simulink model "sm_DynamicCompression"  (R2019b)
settings: Solver=FixedStepDiscrete  StartTime=0.0  StopTime=stop_time  RelTol=1e-3
InitFcn:
  | sm_callback_init
StopFcn:
  | sm_callback_stop
values from neighbouring files (symbols this model uses):
  a = 100*(r^2)    [InitializeCompressionSettings.m]    (also in sm_check_control_signals.m = registers(i).(supplied_fields{j}); sm_check_control_signals_LOCAL_1434.m = registers(i).(supplied_fields{j}))
  B_k_0_init = zeros(1,FIR_0_Uprate)    [sm_callback_init.m]
  B_k_1_init = zeros(1,FIR_0_Uprate)    [sm_callback_init.m]
  B_k_2_init = zeros(1,FIR_0_Uprate)    [sm_callback_init.m]
  B_k_3_init = zeros(1,FIR_0_Uprate)    [sm_callback_init.m]
  B_k_4_init = zeros(1,FIR_0_Uprate)    [sm_callback_init.m]
  B_k_5_init = zeros(1,FIR_0_Uprate)    [sm_callback_init.m]
  calib_bpfs = bpfs    [sm_compression_init.m]
  delayFix = maxDelay-delays    [Initialize_Delay_Values.m]
  F_bits = 28    [TestingLibraryScripts.m]    (also in sm_compression_init.m)
  FIR_0_Size = (ceil(log2(length(calib_bpfs(2:calib_bpfs(1,1)+1 ,1)'))))    [sm_callback_init.m]
  FIR_0_Uprate = 2^FIR_0_Size    [sm_callback_init.m]
  M_bits = 1    [TestingLibraryScripts.m]    (also in sm_compression_init.m = 5)
  M_Bits = M_bits    (= 5)    [sm_compression_init.m]
  mp = sm_init_avalon_signals(mp)    [sm_callback_init.m]
  r_att = nthroot(0.1, s_att)    [sm_compression_init.m]
  r_rel = nthroot(0.1, s_rel)    [sm_compression_init.m]
  recombGain = ones(1,NChans)    [sm_compression_init.m]
  TABLE_SEL_BYPASS_ENABLE = 0    [sm_callback_init.m]
  Ts = mp.Ts    [sm_compression_init.m]
  Ts_system = mp.Ts_system    [sm_compression_init.m]
  W_bits = 32    [TestingLibraryScripts.m]    (also in sm_compression_init.m)
  X_high = 1    [sm_compression_init.m]
undefined symbols (not defined in the file or in its folder): b, c, Gain_Table, ig_eq
libraries: hdlsllib x272, simulink x127, dsphdlfiltering x2
(part 7 of 8)

== matlab function sm_DynamicCompression/dataplane/Avalon Data Processing/Left Channel Processing/recalculate/Nchan_FbankAGC_AID/Compression_1/Compression_Gain_Calc/LogAddressing/MATLAB Function ==
  data: x input; lzc_count output
function lzc_count = fcn(x)
%#codegen

% -- Binary Bisection Tree (Divide & Conquer)
if bitorreduce(x, 40, 21) == 1 %       if ((b39 or b38 or b37 or b36 or b35 or b34 or b33 or b32 or b31 or b30 or b29 or b28 or b27 or b26 or b25 or b24 or b23 or b22 or b21 or b20) = '1') then   -- check bit range [39  20]
    if bitorreduce(x, 40, 31) == 1%             if ((b39 or b38 or b37 or b36 or b35 or b34 or b33 or b32 or b31 or b30) = '1') then   -- check bit range [39  30]
        if bitorreduce(x, 40, 36) == 1%                 if ((b39 or b38 or b37 or b36 or b35) = '1') then   -- check bit range [39  35]
            if bitorreduce(x, 40, 38) == 1%                     if ((b39 or b38 or b37) = '1') then   -- check bit range [39  37]
                if bitorreduce(x, 40, 39) == 1%                         if ((b39 or b38) = '1') then   -- check bit range [39  38]
                    if bitorreduce(x, 40, 40) == 1%                             if (b39 = '1') then   -- [39]
                        lzc_count = fi(0,0,6,0);%                                 lzc_count <= "000000";  -- lzc = 0
                    else%                             else  -- check bit range [38]
                        lzc_count = fi(1,0,6,0);%                                 lzc_count <= "000001";  -- lzc = 1
                    end%                             end if;
                else%                         else  -- check bit range [37]
                    lzc_count = fi(2,0,6,0);%                             lzc_count <= "000010";  -- lzc = 2
                end%                         end if;
            else%                     else  -- check bit range [36  35]
                if bitorreduce(x, 37, 37) == 1%                         if (b36 = '1') then   -- [36]
                    lzc_count = fi(3,0,6,0);%                             lzc_count <= "000011";  -- lzc = 3
                else%                         else  -- check bit range [35]
                    lzc_count = fi(4,0,6,0);%                             lzc_count <= "000100";  -- lzc = 4
                end%                         end if;
            end%                     end if;
        else%                 else  -- check bit range [34  30]
            if bitorreduce(x, 35, 33) == 1%                     if ((b34 or b33 or b32) = '1') then   -- check bit range [34  32]
                if bitorreduce(x, 35, 34) == 1%                         if ((b34 or b33) = '1') then   -- check bit range [34  33]
                    if bitorreduce(x, 35, 35) == 1%                             if (b34 = '1') then   -- [34]
                        lzc_count = fi(5,0,6,0);%                                 lzc_count <= "000101";  -- lzc = 5
                    else%                             else  -- check bit range [33]
                        lzc_count = fi(6,0,6,0);%                                 lzc_count <= "000110";  -- lzc = 6
                    end%                             end if;
                else%                         else  -- check bit range [32]
                    lzc_count = fi(7,0,6,0);%                             lzc_count <= "000111";  -- lzc = 7
                end%                         end if;
            else%                     else  -- check bit range [31  30]
                if bitorreduce(x, 32, 32) == 1%                         if (b31 = '1') then   -- [31]
                    lzc_count = fi(8,0,6,0);%                             lzc_count <= "001000";  -- lzc = 8
                else%                         else  -- check bit range [30]
                    lzc_count = fi(9,0,6,0);%                             lzc_count <= "001001";  -- lzc = 9
                end%                         end if;
            end%                     end if;
        end%                 end if;
    else%             else  -- check bit range [29  20]
        if bitorreduce(x, 30, 26) == 1%                 if ((b29 or b28 or b27 or b26 or b25) = '1') then   -- check bit range [29  25]
            if bitorreduce(x, 30, 28) == 1%                     if ((b29 or b28 or b27) = '1') then   -- check bit range [29  27]
                if bitorreduce(x, 30, 29) == 1%                         if ((b29 or b28) = '1') then   -- check bit range [29  28]
                    if bitorreduce(x, 30, 30) == 1%                             if (b29 = '1') then   -- [29]
                        lzc_count = fi(10,0,6,0);%                                 lzc_count <= "001010";  -- lzc = 10
                    else%                             else  -- check bit range [28]
                        lzc_count = fi(11,0,6,0);%                                 lzc_count <= "001011";  -- lzc = 11
                    end%                             end if;
                else%                         else  -- check bit range [27]
                    lzc_count = fi(12,0,6,0);%                             lzc_count <= "001100";  -- lzc = 12
                end%                         end if;
            else%                     else  -- check bit range [26  25]
                if bitorreduce(x, 27, 27) == 1%                         if (b26 = '1') then   -- [26]
                    lzc_count = fi(13,0,6,0);%                             lzc_count <= "001101";  -- lzc = 13
                else%                         else  -- check bit range [25]
                    lzc_count = fi(14,0,6,0);%                             lzc_count <= "001110";  -- lzc = 14
                end%                         end if;
            end%                     end if;
        else%                 else  -- check bit range [24  20]
            if bitorreduce(x, 25, 23) == 1%                     if ((b24 or b23 or b22) = '1') then   -- check bit range [24  22]
                if bitorreduce(x, 25, 24) == 1%                         if ((b24 or b23) = '1') then   -- check bit range [24  23]
                    if bitorreduce(x, 25, 25) == 1%                             if (b24 = '1') then   -- [24]
                        lzc_count = fi(15,0,6,0);%                                 lzc_count <= "001111";  -- lzc = 15
                    else%                             else  -- check bit range [23]
                        lzc_count = fi(16,0,6,0);%                                 lzc_count <= "010000";  -- lzc = 16
                    end%                             end if;
                else%                         else  -- check bit range [22]
                    lzc_count = fi(17,0,6,0);%                             lzc_count <= "010001";  -- lzc = 17
                end%                         end if;
            else%                     else  -- check bit range [21  20]
                if bitorreduce(x, 22, 22) == 1%                         if (b21 = '1') then   -- [21]
                    lzc_count = fi(18,0,6,0);%                             lzc_count <= "010010";  -- lzc = 18
                else%                         else  -- check bit range [20]
                    lzc_count = fi(19,0,6,0);%                             lzc_count <= "010011";  -- lzc = 19
                end%                         end if;
            end%                     end if;
        end%                 end if;
    end%             end if;
else%         else  -- check bit range [19   0]
    if bitorreduce(x, 20, 11) == 1%             if ((b19 or b18 or b17 or b16 or b15 or b14 or b13 or b12 or b11 or b10) = '1') then   -- check bit range [19  10]
        if bitorreduce(x, 20, 16) == 1%                 if ((b19 or b18 or b17 or b16 or b15) = '1') then   -- check bit range [19  15]
            if bitorreduce(x, 20, 18) == 1%                     if ((b19 or b18 or b17) = '1') then   -- check bit range [19  17]
                if bitorreduce(x, 20, 19) == 1%                         if ((b19 or b18) = '1') then   -- check bit range [19  18]
                    if bitorreduce(x, 20, 20) == 1%                             if (b19 = '1') then   -- [19]
                        lzc_count = fi(20,0,6,0);%                                 lzc_count <= "010100";  -- lzc = 20
                    else%                             else  -- check bit range [18]
                        lzc_count = fi(21,0,6,0);%                                 lzc_count <= "010101";  -- lzc = 21
                    end%                             end if;
                else%                         else  -- check bit range [17]
                    lzc_count = fi(22,0,6,0);%                             lzc_count <= "010110";  -- lzc = 22
                end%                         end if;
            else%                     else  -- check bit range [16  15]
                if bitorreduce(x, 17, 17) == 1%                         if (b16 = '1') then   -- [16]
                    lzc_count = fi(23,0,6,0);%                             lzc_count <= "010111";  -- lzc = 23
                else%                         else  -- check bit range [15]
                    lzc_count = fi(24,0,6,0);%                             lzc_count <= "011000";  -- lzc = 24
                end%                         end if;
            end%                     end if;
        else%                 else  -- check bit range [14  10]
            if bitorreduce(x, 15, 13) == 1%                     if ((b14 or b13 or b12) = '1') then   -- check bit range [14  12]
                if bitorreduce(x, 15, 14) == 1%                         if ((b14 or b13) = '1') then   -- check bit range [14  13]
                    if bitorreduce(x, 15, 15) == 1%                             if (b14 = '1') then   -- [14]
                        lzc_count = fi(25,0,6,0);%                                 lzc_count <= "011001";  -- lzc = 25
                    else%                             else  -- check bit range [13]
                        lzc_count = fi(26,0,6,0);%                                 lzc_count <= "011010";  -- lzc = 26
                    end%                             end if;
                else%                         else  -- check bit range [12]
                    lzc_count = fi(27,0,6,0);%                             lzc_count <= "011011";  -- lzc = 27
                end%                         end if;
            else%                     else  -- check bit range [11  10]
                if bitorreduce(x, 12, 12) == 1%                         if (b11 = '1') then   -- [11]
                    lzc_count = fi(28,0,6,0);%                             lzc_count <= "011100";  -- lzc = 28
                else%                         else  -- check bit range [10]
                    lzc_count = fi(29,0,6,0);%                             lzc_count <= "011101";  -- lzc = 29
                end%                         end if;
            end%                     end if;
        end%                 end if;
    else%             else  -- check bit range [9  0]
        if bitorreduce(x, 10, 6) == 1%                 if ((b9 or b8 or b7 or b6 or b5) = '1') then   -- check bit range [9  5]
            if bitorreduce(x, 10, 9) == 1%                     if ((b9 or b8 or b7) = '1') then   -- check bit range [9  7]
                if bitorreduce(x, 10, 9) == 1%                         if ((b9 or b8) = '1') then   -- check bit range [9  8]
                    if bitorreduce(x, 10, 10) == 1%                             if (b9 = '1') then   -- [9]
                        lzc_count = fi(30,0,6,0);%                                 lzc_count <= "011110";  -- lzc = 30
                    else%                             else  -- check bit range [8]
                        lzc_count = fi(31,0,6,0);%                                 lzc_count <= "011111";  -- lzc = 31
                    end%                             end if;
                else%                         else  -- check bit range [7]
                    lzc_count = fi(32,0,6,0);%                             lzc_count <= "100000";  -- lzc = 32
                end%                         end if;
            else%                     else  -- check bit range [6  5]
                if bitorreduce(x, 7, 7) == 1%                         if (b6 = '1') then   -- [6]
                    lzc_count = fi(33,0,6,0);%                             lzc_count <= "100001";  -- lzc = 33
                else%                         else  -- check bit range [5]
                    lzc_count = fi(34,0,6,0);%                             lzc_count <= "100010";  -- lzc = 34
                end%                         end if;
            end%                     end if;
        else%                 else  -- check bit range [4  0]
            if bitorreduce(x, 5, 3) == 1%                     if ((b4 or b3 or b2) = '1') then   -- check bit range [4  2]
                if bitorreduce(x, 5, 4) == 1%                         if ((b4 or b3) = '1') then   -- check bit range [4  3]
                    if bitorreduce(x, 5, 5) == 1%                             if (b4 = '1') then   -- [4]
                        lzc_count = fi(35,0,6,0);%                                 lzc_count <= "100011";  -- lzc = 35
                    else%                             else  -- check bit range [3]
                        lzc_count = fi(36,0,6,0);%                                 lzc_count <= "100100";  -- lzc = 36
                    end%                             end if;
                else%                         else  -- check bit range [2]
                    lzc_count = fi(37,0,6,0);%                             lzc_count <= "100101";  -- lzc = 37
                end%                         end if;
            else%                     else  -- check bit range [1  0]
                if bitorreduce(x, 2, 2) == 1%                         if (b1 = '1') then   -- [1]
                    lzc_count = fi(38,0,6,0);%                             lzc_count <= "100110";  -- lzc = 38
                else%                         else  -- check bit range [0]
                    lzc_count = fi(39,0,6,0);%                             lzc_count <= "100111";  -- lzc = 39
                end%                         end if;
            end%                     end if;
        end%                 end if;
    end%             end if;
end%         end if;

== matlab function sm_DynamicCompression/dataplane/Avalon Data Processing/Left Channel Processing/recalculate/Nchan_FbankAGC_AID/Compression_3/Compression_Gain_Calc/LogAddressing/MATLAB Function ==
  data: x input; lzc_count output
function lzc_count = fcn(x)
%#codegen

% -- Binary Bisection Tree (Divide & Conquer)
if bitorreduce(x, 40, 21) == 1 %       if ((b39 or b38 or b37 or b36 or b35 or b34 or b33 or b32 or b31 or b30 or b29 or b28 or b27 or b26 or b25 or b24 or b23 or b22 or b21 or b20) = '1') then   -- check bit range [39  20]
    if bitorreduce(x, 40, 31) == 1%             if ((b39 or b38 or b37 or b36 or b35 or b34 or b33 or b32 or b31 or b30) = '1') then   -- check bit range [39  30]
        if bitorreduce(x, 40, 36) == 1%                 if ((b39 or b38 or b37 or b36 or b35) = '1') then   -- check bit range [39  35]
            if bitorreduce(x, 40, 38) == 1%                     if ((b39 or b38 or b37) = '1') then   -- check bit range [39  37]
                if bitorreduce(x, 40, 39) == 1%                         if ((b39 or b38) = '1') then   -- check bit range [39  38]
                    if bitorreduce(x, 40, 40) == 1%                             if (b39 = '1') then   -- [39]
                        lzc_count = fi(0,0,6,0);%                                 lzc_count <= "000000";  -- lzc = 0
                    else%                             else  -- check bit range [38]
                        lzc_count = fi(1,0,6,0);%                                 lzc_count <= "000001";  -- lzc = 1
                    end%                             end if;
                else%                         else  -- check bit range [37]
                    lzc_count = fi(2,0,6,0);%                             lzc_count <= "000010";  -- lzc = 2
                end%                         end if;
            else%                     else  -- check bit range [36  35]
                if bitorreduce(x, 37, 37) == 1%                         if (b36 = '1') then   -- [36]
                    lzc_count = fi(3,0,6,0);%                             lzc_count <= "000011";  -- lzc = 3
                else%                         else  -- check bit range [35]
                    lzc_count = fi(4,0,6,0);%                             lzc_count <= "000100";  -- lzc = 4
                end%                         end if;
            end%                     end if;
        else%                 else  -- check bit range [34  30]
            if bitorreduce(x, 35, 33) == 1%                     if ((b34 or b33 or b32) = '1') then   -- check bit range [34  32]
                if bitorreduce(x, 35, 34) == 1%                         if ((b34 or b33) = '1') then   -- check bit range [34  33]
                    if bitorreduce(x, 35, 35) == 1%                             if (b34 = '1') then   -- [34]
                        lzc_count = fi(5,0,6,0);%                                 lzc_count <= "000101";  -- lzc = 5
                    else%                             else  -- check bit range [33]
                        lzc_count = fi(6,0,6,0);%                                 lzc_count <= "000110";  -- lzc = 6
                    end%                             end if;
                else%                         else  -- check bit range [32]
                    lzc_count = fi(7,0,6,0);%                             lzc_count <= "000111";  -- lzc = 7
                end%                         end if;
            else%                     else  -- check bit range [31  30]
                if bitorreduce(x, 32, 32) == 1%                         if (b31 = '1') then   -- [31]
                    lzc_count = fi(8,0,6,0);%                             lzc_count <= "001000";  -- lzc = 8
                else%                         else  -- check bit range [30]
                    lzc_count = fi(9,0,6,0);%                             lzc_count <= "001001";  -- lzc = 9
                end%                         end if;
            end%                     end if;
        end%                 end if;
    else%             else  -- check bit range [29  20]
        if bitorreduce(x, 30, 26) == 1%                 if ((b29 or b28 or b27 or b26 or b25) = '1') then   -- check bit range [29  25]
            if bitorreduce(x, 30, 28) == 1%                     if ((b29 or b28 or b27) = '1') then   -- check bit range [29  27]
                if bitorreduce(x, 30, 29) == 1%                         if ((b29 or b28) = '1') then   -- check bit range [29  28]
                    if bitorreduce(x, 30, 30) == 1%                             if (b29 = '1') then   -- [29]
                        lzc_count = fi(10,0,6,0);%                                 lzc_count <= "001010";  -- lzc = 10
                    else%                             else  -- check bit range [28]
                        lzc_count = fi(11,0,6,0);%                                 lzc_count <= "001011";  -- lzc = 11
                    end%                             end if;
                else%                         else  -- check bit range [27]
                    lzc_count = fi(12,0,6,0);%                             lzc_count <= "001100";  -- lzc = 12
                end%                         end if;
            else%                     else  -- check bit range [26  25]
                if bitorreduce(x, 27, 27) == 1%                         if (b26 = '1') then   -- [26]
                    lzc_count = fi(13,0,6,0);%                             lzc_count <= "001101";  -- lzc = 13
                else%                         else  -- check bit range [25]
                    lzc_count = fi(14,0,6,0);%                             lzc_count <= "001110";  -- lzc = 14
                end%                         end if;
            end%                     end if;
        else%                 else  -- check bit range [24  20]
            if bitorreduce(x, 25, 23) == 1%                     if ((b24 or b23 or b22) = '1') then   -- check bit range [24  22]
                if bitorreduce(x, 25, 24) == 1%                         if ((b24 or b23) = '1') then   -- check bit range [24  23]
                    if bitorreduce(x, 25, 25) == 1%                             if (b24 = '1') then   -- [24]
                        lzc_count = fi(15,0,6,0);%                                 lzc_count <= "001111";  -- lzc = 15
                    else%                             else  -- check bit range [23]
                        lzc_count = fi(16,0,6,0);%                                 lzc_count <= "010000";  -- lzc = 16
                    end%                             end if;
                else%                         else  -- check bit range [22]
                    lzc_count = fi(17,0,6,0);%                             lzc_count <= "010001";  -- lzc = 17
                end%                         end if;
            else%                     else  -- check bit range [21  20]
                if bitorreduce(x, 22, 22) == 1%                         if (b21 = '1') then   -- [21]
                    lzc_count = fi(18,0,6,0);%                             lzc_count <= "010010";  -- lzc = 18
                else%                         else  -- check bit range [20]
                    lzc_count = fi(19,0,6,0);%                             lzc_count <= "010011";  -- lzc = 19
                end%                         end if;
            end%                     end if;
        end%                 end if;
    end%             end if;
else%         else  -- check bit range [19   0]
    if bitorreduce(x, 20, 11) == 1%             if ((b19 or b18 or b17 or b16 or b15 or b14 or b13 or b12 or b11 or b10) = '1') then   -- check bit range [19  10]
        if bitorreduce(x, 20, 16) == 1%                 if ((b19 or b18 or b17 or b16 or b15) = '1') then   -- check bit range [19  15]
            if bitorreduce(x, 20, 18) == 1%                     if ((b19 or b18 or b17) = '1') then   -- check bit range [19  17]
                if bitorreduce(x, 20, 19) == 1%                         if ((b19 or b18) = '1') then   -- check bit range [19  18]
                    if bitorreduce(x, 20, 20) == 1%                             if (b19 = '1') then   -- [19]
                        lzc_count = fi(20,0,6,0);%                                 lzc_count <= "010100";  -- lzc = 20
                    else%                             else  -- check bit range [18]
                        lzc_count = fi(21,0,6,0);%                                 lzc_count <= "010101";  -- lzc = 21
                    end%                             end if;
                else%                         else  -- check bit range [17]
                    lzc_count = fi(22,0,6,0);%                             lzc_count <= "010110";  -- lzc = 22
                end%                         end if;
            else%                     else  -- check bit range [16  15]
                if bitorreduce(x, 17, 17) == 1%                         if (b16 = '1') then   -- [16]
                    lzc_count = fi(23,0,6,0);%                             lzc_count <= "010111";  -- lzc = 23
                else%                         else  -- check bit range [15]
                    lzc_count = fi(24,0,6,0);%                             lzc_count <= "011000";  -- lzc = 24
                end%                         end if;
            end%                     end if;
        else%                 else  -- check bit range [14  10]
            if bitorreduce(x, 15, 13) == 1%                     if ((b14 or b13 or b12) = '1') then   -- check bit range [14  12]
                if bitorreduce(x, 15, 14) == 1%                         if ((b14 or b13) = '1') then   -- check bit range [14  13]
                    if bitorreduce(x, 15, 15) == 1%                             if (b14 = '1') then   -- [14]
                        lzc_count = fi(25,0,6,0);%                                 lzc_count <= "011001";  -- lzc = 25
                    else%                             else  -- check bit range [13]
                        lzc_count = fi(26,0,6,0);%                                 lzc_count <= "011010";  -- lzc = 26
                    end%                             end if;
                else%                         else  -- check bit range [12]
                    lzc_count = fi(27,0,6,0);%                             lzc_count <= "011011";  -- lzc = 27
                end%                         end if;
            else%                     else  -- check bit range [11  10]
                if bitorreduce(x, 12, 12) == 1%                         if (b11 = '1') then   -- [11]
                    lzc_count = fi(28,0,6,0);%                             lzc_count <= "011100";  -- lzc = 28
                else%                         else  -- check bit range [10]
                    lzc_count = fi(29,0,6,0);%                             lzc_count <= "011101";  -- lzc = 29
                end%                         end if;
            end%                     end if;
        end%                 end if;
    else%             else  -- check bit range [9  0]
        if bitorreduce(x, 10, 6) == 1%                 if ((b9 or b8 or b7 or b6 or b5) = '1') then   -- check bit range [9  5]
            if bitorreduce(x, 10, 9) == 1%                     if ((b9 or b8 or b7) = '1') then   -- check bit range [9  7]
                if bitorreduce(x, 10, 9) == 1%                         if ((b9 or b8) = '1') then   -- check bit range [9  8]
                    if bitorreduce(x, 10, 10) == 1%                             if (b9 = '1') then   -- [9]
                        lzc_count = fi(30,0,6,0);%                                 lzc_count <= "011110";  -- lzc = 30
                    else%                             else  -- check bit range [8]
                        lzc_count = fi(31,0,6,0);%                                 lzc_count <= "011111";  -- lzc = 31
                    end%                             end if;
                else%                         else  -- check bit range [7]
                    lzc_count = fi(32,0,6,0);%                             lzc_count <= "100000";  -- lzc = 32
                end%                         end if;
            else%                     else  -- check bit range [6  5]
                if bitorreduce(x, 7, 7) == 1%                         if (b6 = '1') then   -- [6]
                    lzc_count = fi(33,0,6,0);%                             lzc_count <= "100001";  -- lzc = 33
                else%                         else  -- check bit range [5]
                    lzc_count = fi(34,0,6,0);%                             lzc_count <= "100010";  -- lzc = 34
                end%                         end if;
            end%                     end if;
        else%                 else  -- check bit range [4  0]
            if bitorreduce(x, 5, 3) == 1%                     if ((b4 or b3 or b2) = '1') then   -- check bit range [4  2]
                if bitorreduce(x, 5, 4) == 1%                         if ((b4 or b3) = '1') then   -- check bit range [4  3]
                    if bitorreduce(x, 5, 5) == 1%                             if (b4 = '1') then   -- [4]
                        lzc_count = fi(35,0,6,0);%                                 lzc_count <= "100011";  -- lzc = 35
                    else%                             else  -- check bit range [3]
                        lzc_count = fi(36,0,6,0);%                                 lzc_count <= "100100";  -- lzc = 36
                    end%                             end if;
                else%                         else  -- check bit range [2]
                    lzc_count = fi(37,0,6,0);%                             lzc_count <= "100101";  -- lzc = 37
                end%                         end if;
            else%                     else  -- check bit range [1  0]
                if bitorreduce(x, 2, 2) == 1%                         if (b1 = '1') then   -- [1]
                    lzc_count = fi(38,0,6,0);%                             lzc_count <= "100110";  -- lzc = 38
                else%                         else  -- check bit range [0]
                    lzc_count = fi(39,0,6,0);%                             lzc_count <= "100111";  -- lzc = 39
                end%                         end if;
            end%                     end if;
        end%                 end if;
    end%             end if;
end%         end if;

== matlab function sm_DynamicCompression/dataplane/Avalon Data Processing/Left Channel Processing/recalculate/Nchan_FbankAGC_AID/Compression_4/Compression_Gain_Calc/LogAddressing/MATLAB Function ==
  data: x input; lzc_count output
function lzc_count = fcn(x)
%#codegen

% -- Binary Bisection Tree (Divide & Conquer)
if bitorreduce(x, 40, 21) == 1 %       if ((b39 or b38 or b37 or b36 or b35 or b34 or b33 or b32 or b31 or b30 or b29 or b28 or b27 or b26 or b25 or b24 or b23 or b22 or b21 or b20) = '1') then   -- check bit range [39  20]
    if bitorreduce(x, 40, 31) == 1%             if ((b39 or b38 or b37 or b36 or b35 or b34 or b33 or b32 or b31 or b30) = '1') then   -- check bit range [39  30]
        if bitorreduce(x, 40, 36) == 1%                 if ((b39 or b38 or b37 or b36 or b35) = '1') then   -- check bit range [39  35]
            if bitorreduce(x, 40, 38) == 1%                     if ((b39 or b38 or b37) = '1') then   -- check bit range [39  37]
                if bitorreduce(x, 40, 39) == 1%                         if ((b39 or b38) = '1') then   -- check bit range [39  38]
                    if bitorreduce(x, 40, 40) == 1%                             if (b39 = '1') then   -- [39]
                        lzc_count = fi(0,0,6,0);%                                 lzc_count <= "000000";  -- lzc = 0
                    else%                             else  -- check bit range [38]
                        lzc_count = fi(1,0,6,0);%                                 lzc_count <= "000001";  -- lzc = 1
                    end%                             end if;
                else%                         else  -- check bit range [37]
                    lzc_count = fi(2,0,6,0);%                             lzc_count <= "000010";  -- lzc = 2
                end%                         end if;
            else%                     else  -- check bit range [36  35]
                if bitorreduce(x, 37, 37) == 1%                         if (b36 = '1') then   -- [36]
                    lzc_count = fi(3,0,6,0);%                             lzc_count <= "000011";  -- lzc = 3
                else%                         else  -- check bit range [35]
                    lzc_count = fi(4,0,6,0);%                             lzc_count <= "000100";  -- lzc = 4
                end%                         end if;
            end%                     end if;
        else%                 else  -- check bit range [34  30]
            if bitorreduce(x, 35, 33) == 1%                     if ((b34 or b33 or b32) = '1') then   -- check bit range [34  32]
                if bitorreduce(x, 35, 34) == 1%                         if ((b34 or b33) = '1') then   -- check bit range [34  33]
                    if bitorreduce(x, 35, 35) == 1%                             if (b34 = '1') then   -- [34]
                        lzc_count = fi(5,0,6,0);%                                 lzc_count <= "000101";  -- lzc = 5
                    else%                             else  -- check bit range [33]
                        lzc_count = fi(6,0,6,0);%                                 lzc_count <= "000110";  -- lzc = 6
                    end%                             end if;
                else%                         else  -- check bit range [32]
                    lzc_count = fi(7,0,6,0);%                             lzc_count <= "000111";  -- lzc = 7
                end%                         end if;
            else%                     else  -- check bit range [31  30]
                if bitorreduce(x, 32, 32) == 1%                         if (b31 = '1') then   -- [31]
                    lzc_count = fi(8,0,6,0);%                             lzc_count <= "001000";  -- lzc = 8
                else%                         else  -- check bit range [30]
                    lzc_count = fi(9,0,6,0);%                             lzc_count <= "001001";  -- lzc = 9
                end%                         end if;
            end%                     end if;
        end%                 end if;
    else%             else  -- check bit range [29  20]
        if bitorreduce(x, 30, 26) == 1%                 if ((b29 or b28 or b27 or b26 or b25) = '1') then   -- check bit range [29  25]
            if bitorreduce(x, 30, 28) == 1%                     if ((b29 or b28 or b27) = '1') then   -- check bit range [29  27]
                if bitorreduce(x, 30, 29) == 1%                         if ((b29 or b28) = '1') then   -- check bit range [29  28]
                    if bitorreduce(x, 30, 30) == 1%                             if (b29 = '1') then   -- [29]
                        lzc_count = fi(10,0,6,0);%                                 lzc_count <= "001010";  -- lzc = 10
                    else%                             else  -- check bit range [28]
                        lzc_count = fi(11,0,6,0);%                                 lzc_count <= "001011";  -- lzc = 11
                    end%                             end if;
                else%                         else  -- check bit range [27]
                    lzc_count = fi(12,0,6,0);%                             lzc_count <= "001100";  -- lzc = 12
                end%                         end if;
            else%                     else  -- check bit range [26  25]
                if bitorreduce(x, 27, 27) == 1%                         if (b26 = '1') then   -- [26]
                    lzc_count = fi(13,0,6,0);%                             lzc_count <= "001101";  -- lzc = 13
                else%                         else  -- check bit range [25]
                    lzc_count = fi(14,0,6,0);%                             lzc_count <= "001110";  -- lzc = 14
                end%                         end if;
            end%                     end if;
        else%                 else  -- check bit range [24  20]
            if bitorreduce(x, 25, 23) == 1%                     if ((b24 or b23 or b22) = '1') then   -- check bit range [24  22]
                if bitorreduce(x, 25, 24) == 1%                         if ((b24 or b23) = '1') then   -- check bit range [24  23]
                    if bitorreduce(x, 25, 25) == 1%                             if (b24 = '1') then   -- [24]
                        lzc_count = fi(15,0,6,0);%                                 lzc_count <= "001111";  -- lzc = 15
                    else%                             else  -- check bit range [23]
                        lzc_count = fi(16,0,6,0);%                                 lzc_count <= "010000";  -- lzc = 16
                    end%                             end if;
                else%                         else  -- check bit range [22]
                    lzc_count = fi(17,0,6,0);%                             lzc_count <= "010001";  -- lzc = 17
                end%                         end if;
            else%                     else  -- check bit range [21  20]
                if bitorreduce(x, 22, 22) == 1%                         if (b21 = '1') then   -- [21]
                    lzc_count = fi(18,0,6,0);%                             lzc_count <= "010010";  -- lzc = 18
                else%                         else  -- check bit range [20]
                    lzc_count = fi(19,0,6,0);%                             lzc_count <= "010011";  -- lzc = 19
                end%                         end if;
            end%                     end if;
        end%                 end if;
    end%             end if;
else%         else  -- check bit range [19   0]
    if bitorreduce(x, 20, 11) == 1%             if ((b19 or b18 or b17 or b16 or b15 or b14 or b13 or b12 or b11 or b10) = '1') then   -- check bit range [19  10]
        if bitorreduce(x, 20, 16) == 1%                 if ((b19 or b18 or b17 or b16 or b15) = '1') then   -- check bit range [19  15]
            if bitorreduce(x, 20, 18) == 1%                     if ((b19 or b18 or b17) = '1') then   -- check bit range [19  17]
                if bitorreduce(x, 20, 19) == 1%                         if ((b19 or b18) = '1') then   -- check bit range [19  18]
                    if bitorreduce(x, 20, 20) == 1%                             if (b19 = '1') then   -- [19]
                        lzc_count = fi(20,0,6,0);%                                 lzc_count <= "010100";  -- lzc = 20
                    else%                             else  -- check bit range [18]
                        lzc_count = fi(21,0,6,0);%                                 lzc_count <= "010101";  -- lzc = 21
                    end%                             end if;
                else%                         else  -- check bit range [17]
                    lzc_count = fi(22,0,6,0);%                             lzc_count <= "010110";  -- lzc = 22
                end%                         end if;
            else%                     else  -- check bit range [16  15]
                if bitorreduce(x, 17, 17) == 1%                         if (b16 = '1') then   -- [16]
                    lzc_count = fi(23,0,6,0);%                             lzc_count <= "010111";  -- lzc = 23
                else%                         else  -- check bit range [15]
                    lzc_count = fi(24,0,6,0);%                             lzc_count <= "011000";  -- lzc = 24
                end%                         end if;
            end%                     end if;
        else%                 else  -- check bit range [14  10]
            if bitorreduce(x, 15, 13) == 1%                     if ((b14 or b13 or b12) = '1') then   -- check bit range [14  12]
                if bitorreduce(x, 15, 14) == 1%                         if ((b14 or b13) = '1') then   -- check bit range [14  13]
                    if bitorreduce(x, 15, 15) == 1%                             if (b14 = '1') then   -- [14]
                        lzc_count = fi(25,0,6,0);%                                 lzc_count <= "011001";  -- lzc = 25
                    else%                             else  -- check bit range [13]
                        lzc_count = fi(26,0,6,0);%                                 lzc_count <= "011010";  -- lzc = 26
                    end%                             end if;
                else%                         else  -- check bit range [12]
                    lzc_count = fi(27,0,6,0);%                             lzc_count <= "011011";  -- lzc = 27
                end%                         end if;
            else%                     else  -- check bit range [11  10]
                if bitorreduce(x, 12, 12) == 1%                         if (b11 = '1') then   -- [11]
                    lzc_count = fi(28,0,6,0);%                             lzc_count <= "011100";  -- lzc = 28
                else%                         else  -- check bit range [10]
                    lzc_count = fi(29,0,6,0);%                             lzc_count <= "011101";  -- lzc = 29
                end%                         end if;
            end%                     end if;
        end%                 end if;
    else%             else  -- check bit range [9  0]
        if bitorreduce(x, 10, 6) == 1%                 if ((b9 or b8 or b7 or b6 or b5) = '1') then   -- check bit range [9  5]
            if bitorreduce(x, 10, 9) == 1%                     if ((b9 or b8 or b7) = '1') then   -- check bit range [9  7]
                if bitorreduce(x, 10, 9) == 1%                         if ((b9 or b8) = '1') then   -- check bit range [9  8]
                    if bitorreduce(x, 10, 10) == 1%                             if (b9 = '1') then   -- [9]
                        lzc_count = fi(30,0,6,0);%                                 lzc_count <= "011110";  -- lzc = 30
                    else%                             else  -- check bit range [8]
                        lzc_count = fi(31,0,6,0);%                                 lzc_count <= "011111";  -- lzc = 31
                    end%                             end if;
                else%                         else  -- check bit range [7]
                    lzc_count = fi(32,0,6,0);%                             lzc_count <= "100000";  -- lzc = 32
                end%                         end if;
            else%                     else  -- check bit range [6  5]
                if bitorreduce(x, 7, 7) == 1%                         if (b6 = '1') then   -- [6]
                    lzc_count = fi(33,0,6,0);%                             lzc_count <= "100001";  -- lzc = 33
                else%                         else  -- check bit range [5]
                    lzc_count = fi(34,0,6,0);%                             lzc_count <= "100010";  -- lzc = 34
                end%                         end if;
            end%                     end if;
        else%                 else  -- check bit range [4  0]
            if bitorreduce(x, 5, 3) == 1%                     if ((b4 or b3 or b2) = '1') then   -- check bit range [4  2]
                if bitorreduce(x, 5, 4) == 1%                         if ((b4 or b3) = '1') then   -- check bit range [4  3]
                    if bitorreduce(x, 5, 5) == 1%                             if (b4 = '1') then   -- [4]
                        lzc_count = fi(35,0,6,0);%                                 lzc_count <= "100011";  -- lzc = 35
                    else%                             else  -- check bit range [3]
                        lzc_count = fi(36,0,6,0);%                                 lzc_count <= "100100";  -- lzc = 36
                    end%                             end if;
                else%                         else  -- check bit range [2]
                    lzc_count = fi(37,0,6,0);%                             lzc_count <= "100101";  -- lzc = 37
                end%                         end if;
            else%                     else  -- check bit range [1  0]
                if bitorreduce(x, 2, 2) == 1%                         if (b1 = '1') then   -- [1]
                    lzc_count = fi(38,0,6,0);%                             lzc_count <= "100110";  -- lzc = 38
                else%                         else  -- check bit range [0]
                    lzc_count = fi(39,0,6,0);%                             lzc_count <= "100111";  -- lzc = 39
                end%                         end if;
            end%                     end if;
        end%                 end if;
    end%             end if;
end%         end if;
